simulink model "keshestatefeedback"  (R2017a)
settings: Solver=VariableStepAuto  StartTime=0.0  StopTime=10  MaxStep=0.01  RelTol=1e-3
settings Model: Creator=adi  LastModifiedBy=adi

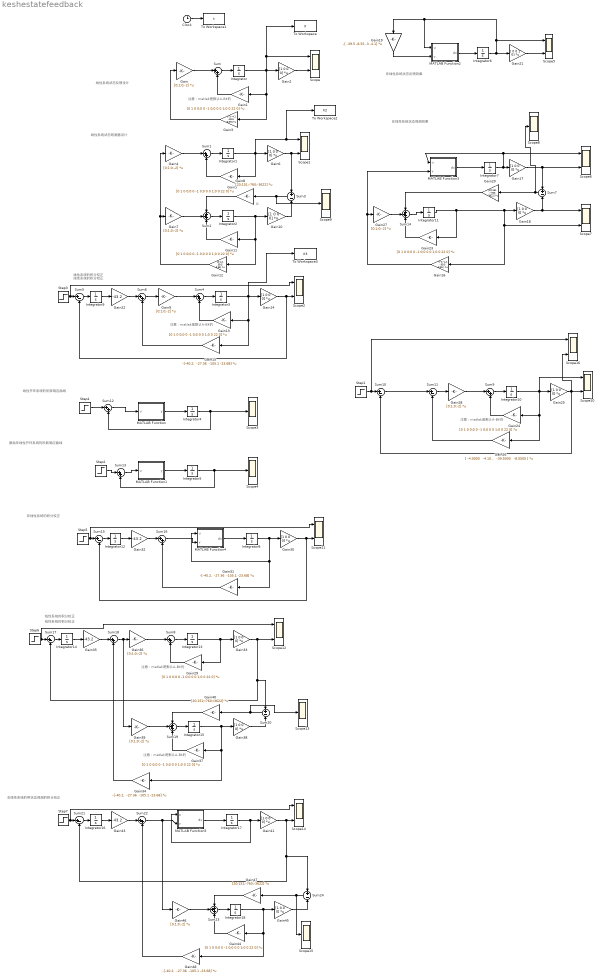
== system keshestatefeedback ==
  note: 非线性系统的积分校正
  note: 线性系统的积分校正
  note: G
  note: 线性系统状态反馈设计
  note: 线性开环系统的阶跃响应曲线
  note: 注意：matlab是默认A-BK的
  note: 注意：matlab是默认A-BK的
  note: 原始非线性开环系统的阶跃响应曲线
  note: 非线性系统状态反馈效果
  note: 非线性系统状态观测效果
  note: 线性系统状态观测器设计
  note: 注意：matlab是默认A-BK的
  note: 线性系统的积分校正
  note: 线性系统的积分校正
  note: 注意：matlab是默认A-BK的
  note: 线性系统的积分校正
  note: 注意：matlab是默认A-BK的
  note: 非线性系统的带状态观测的积分校正
  Clock : Clock
  Gain{,4,7,9,27..28,36,39,46} (9 alike) : Gain  Gain=[0;1;0;-2]  Multiplication=Matrix(K*u)
  Gain{1,5,11,13,23..24,29,37,44} (9 alike) : Gain  Gain=[0 1 0 0;0 0 -1 0;0 0 0 1;0 0 22 0]  Multiplication=Matrix(K*u)
  Gain{2,6,10,14,17..18,25,30,33,38,41,45} (12 alike) : Gain  Gain=[1 0 0 0]  Multiplication=Matrix(K*u)
  Gain12 : Gain  Gain=[3 4.1 39.5 8.55]  Multiplication=Matrix(K*u)
  Gain{15,31,34,48} (4 alike) : Gain  Gain="-[-40.2,  -27.36  -105.1 -23.68]"  Multiplication=Matrix(K*u)
  Gain16 : Gain  Gain="-[-3 -4.1 -39.5  -8.55 ]"  Multiplication=Matrix(K*u)
  Gain19 : Gain  Gain=-[ -39.5 -8.55 -3 -4.1]  Multiplication=Matrix(K*u)
  Gain20 : Gain  Gain="[20;151 ;-760;  -3622]"  Multiplication=Matrix(K*u)
  Gain21 : Gain  Gain=[ 0 0 1 0]  Multiplication=Matrix(K*u)
  Gain{22,32,35,43} (4 alike) : Gain  Gain=-43.2
  Gain26 : Gain  Gain=|  Multiplication=Matrix(K*u)
      | [ -4.0000   -4.1000  -39.5000   -8.5500
      | ]
  Gain3 : Gain  Gain=-[-3 -4.1 -39.5 -8.55]  Multiplication=Matrix(K*u)
  Gain40 : Gain  Gain=[20;151;-760;-3622]  Multiplication=Matrix(K*u)
  Gain47 : Gain  Gain=[20;151;-760;-3622]  Multiplication=Matrix(K*u)
  Gain8 : Gain  Gain=[20;151;-760;-3622]  Multiplication=Matrix(K*u)
  Integrator : Integrator  InitialCondition=[0.1 0 0 0]
  Integrator1 : Integrator  InitialCondition=[0.1 0 0 0]
  Integrator{3..5,8,10,13,15,17..18} (9 alike) : Integrator  InitialCondition=[0 0 0 0]
  Integrator11 : Integrator  InitialCondition=[0 0 0.1 0]
  Integrator{9,12,14,16} (4 alike) : Integrator
  Integrator2 : Integrator  InitialCondition=[0.001 0 0 0]
  Integrator6 : Integrator  InitialCondition=[0.1 0 0 0]
  Integrator7 : Integrator  InitialCondition=[0 0 0.1 0]
  MATLAB Function : MATLAB Function  TreatAsAtomicUnit=on
  MATLAB Function1 : MATLAB Function  TreatAsAtomicUnit=on
  MATLAB Function2 : MATLAB Function  TreatAsAtomicUnit=on
  MATLAB Function3 : MATLAB Function  TreatAsAtomicUnit=on
  MATLAB Function4 : MATLAB Function  TreatAsAtomicUnit=on
  MATLAB Function5 : MATLAB Function  TreatAsAtomicUnit=on
  Scope{,1..2,5..7,10..12,14,16} (11 alike) : Scope  NumInputPorts=2
  Scope{3..4,8..9,13,15} (6 alike) : Scope
  Step{1,3,5..7} (5 alike) : Step  After=0.1  SampleTime=0
  Step2 : Step  SampleTime=0
  Step4 : Step  SampleTime=0
  Sum{,1,4,6,8..9,12..13,16,18,22} (11 alike) : Sum  Inputs=|++
  Sum{5,10..11,15,17,21} (6 alike) : Sum  Inputs=|+-
  Sum{2,14,19,23} (4 alike) : Sum  Inputs=+++
  Sum{3,7,20,24} (4 alike) : Sum  Inputs=+-
  To Workspace : ToWorkspace  VariableName=X  SaveFormat=Structure With Time  SampleTime=-1
  To Workspace1 : ToWorkspace  VariableName=t  SaveFormat=Structure With Time  SampleTime=-1
  To Workspace2 : ToWorkspace  VariableName=X2  SaveFormat=Structure With Time  SampleTime=-1
  To Workspace3 : ToWorkspace  VariableName=X3  SaveFormat=Structure With Time  SampleTime=-1
  wires:
  Gain/1 -> Sum/1
  Sum/1 -> Integrator/1
  Integrator/1 -> To Workspace/1, Scope/1, Gain3/1, Gain1/1, Gain2/1
  Gain1/1 -> Sum/2
  Gain2/1 -> Scope/2
  Gain3/1 -> Gain/1
  Gain4/1 -> Sum1/1
  Sum1/1 -> Integrator1/1
  Gain5/1 -> Sum1/2
  Gain6/1 -> Sum3/1, Scope1/2
  Gain7/1 -> Sum2/2
  Sum2/1 -> Integrator2/1
  Gain10/1 -> Sum3/2
  Sum3/1 -> Scope9/1, Gain8/1
  Gain8/1 -> Sum2/1
  Gain11/1 -> Sum2/3
  Integrator2/1 -> Gain10/1, Gain12/1, Gain11/1
  Sum4/1 -> Integrator3/1
  Gain13/1 -> Sum4/2
  Gain15/1 -> Sum6/2
  Sum6/1 -> Gain9/1
  Gain12/1 -> Gain7/1, Gain4/1
  Clock/1 -> To Workspace1/1
  Integrator1/1 -> To Workspace2/1, Scope1/1, Gain5/1, Gain6/1
  Integrator3/1 -> To Workspace3/1, Gain15/1, Gain13/1, Gain14/1
  MATLAB Function/1(y) -> Integrator4/1
  Integrator4/1 -> Sum12/2, Scope3/1
  Integrator5/1 -> Sum13/2, Scope4/1
  MATLAB Function1/1(y) -> Integrator5/1
  MATLAB Function3/1(dx) -> Integrator7/1
  Integrator11/1 -> Gain23/1, Scope7/2, Gain16/1, Gain18/1
  Integrator7/1 -> MATLAB Function3/1(u), Scope6/1, Gain17/1
  Gain17/1 -> Sum7/1, Scope6/2
  Gain18/1 -> Sum7/2, Scope7/1
  Sum7/1 -> Scope8/1, Gain20/1
  Gain16/1 -> Gain27/1, MATLAB Function3/2(v)
  Integrator6/1 -> Gain21/1, Scope5/1, MATLAB Function2/1(u), Gain19/1
  MATLAB Function2/1(dx) -> Integrator6/1
  Gain19/1 -> MATLAB Function2/2(v)
  Gain21/1 -> Scope5/2
  Integrator9/1 -> Gain22/1
  Gain22/1 -> Sum6/1
  Gain25/1 -> Scope16/2, Sum10/2, Scope10/2
  Gain24/1 -> Sum9/2
  Sum9/1 -> Integrator10/1
  Integrator10/1 -> Scope10/1, Gain26/1, Gain24/1, Gain25/1
  Sum11/1 -> Gain28/1
  Gain28/1 -> Sum9/1
  Step1/1 -> Scope16/1, Sum10/1
  Gain26/1 -> Sum11/2
  Sum10/1 -> Sum11/1
  Sum5/1 -> Integrator9/1
  Step3/1 -> Scope2/1, Sum5/1
  Gain14/1 -> Sum5/2, Scope2/2
  Step4/1 -> Sum12/1
  Sum12/1 -> MATLAB Function/1(u)
  Gain9/1 -> Sum4/1
  Step2/1 -> Sum13/1
  Sum13/1 -> MATLAB Function1/1(u)
  Sum14/1 -> Integrator11/1
  Gain23/1 -> Sum14/3
  Gain27/1 -> Sum14/2
  Gain20/1 -> Sum14/1
  Integrator12/1 -> Gain32/1
  Gain30/1 -> Sum15/2, Scope11/2
  Gain31/1 -> Sum16/2
  Gain32/1 -> Sum16/1
  Step5/1 -> Scope11/1, Sum15/1
  Sum15/1 -> Integrator12/1
  Sum16/1 -> MATLAB Function4/2(v)
  MATLAB Function4/1(dx) -> Integrator8/1
  Integrator8/1 -> Gain31/1, MATLAB Function4/1(u), Gain30/1
  Sum8/1 -> Integrator13/1
  Gain29/1 -> Sum8/2
  Gain36/1 -> Sum8/1
  Integrator14/1 -> Gain35/1
  Gain34/1 -> Sum18/2
  Gain35/1 -> Sum18/1
  Integrator13/1 -> Gain29/1, Gain33/1
  Step6/1 -> Scope12/1, Sum17/1
  Sum18/1 -> Gain39/1, Gain36/1
  Sum17/1 -> Integrator14/1
  Integrator15/1 -> Gain34/1, Gain37/1, Gain38/1
  Sum19/1 -> Integrator15/1
  Gain39/1 -> Sum19/2
  Gain37/1 -> Sum19/3
  Gain33/1 -> Sum20/1, Sum17/2, Scope12/2
  Gain38/1 -> Sum20/2
  Sum20/1 -> Scope13/1, Gain40/1
  Gain40/1 -> Sum19/1
  Integrator17/1 -> MATLAB Function5/1(u), Gain41/1
  MATLAB Function5/1(dx) -> Integrator17/1
  Sum22/1 -> Gain46/1, MATLAB Function5/2(v)
  Step7/1 -> Scope14/1, Sum21/1
  Sum21/1 -> Integrator16/1
  Integrator16/1 -> Gain43/1
  Gain43/1 -> Sum22/1
  Sum24/1 -> Gain47/1, Scope15/1
  Gain44/1 -> Sum23/3
  Gain45/1 -> Sum24/2
  Sum23/1 -> Integrator18/1
  Gain47/1 -> Sum23/1
  Integrator18/1 -> Gain48/1, Gain44/1, Gain45/1
  Gain46/1 -> Sum23/2
  Gain41/1 -> Sum24/1, Sum21/2, Scope14/2
  Gain48/1 -> Sum22/2

== matlab function keshestatefeedback/MATLAB Function1 ==
  data: u input; y output
function y = fcn(u)
M=1;m=0.1;l=0.5;g=9.8;v=0;
dx1 = u(2);
dx2 = (v*cos(u(1))-(M+m)*g*sin(u(1))+m*l*sin(u(1))*cos(u(1)*u(2)*u(2)))/(m*l*cos(u(1))*cos(u(1))-(M+m)*l);
dx3 = u(4);
dx4 = (v+m*l*sin(u(1)*u(2)*u(2))-m*g*cos(u(1))*sin(u(1)))/(M+m-m*cos(u(1))*cos(u(1)));
y = [dx1;dx2;dx3;dx4];

== matlab function keshestatefeedback/MATLAB Function ==
  data: u input; y output
function y = fcn(u)
M=1;m=0.1;l=0.5;g=9.8;v=0;
dx1 = u(2);
dx2 = (-1*m*g/M)*u(3)+(1/M)*v;
dx3 = u(4);
dx4 = ((M+m)*g/M/l)*u(3)-(1/M/l)*v;
y = [dx1;dx2;dx3;dx4];

== matlab function keshestatefeedback/MATLAB Function2 ==
  data: dx output; u input; v input
function dx = fcn(u,v)
M=1;m=0.1;l=0.5;g=10;
%v=0;
dx1 = u(2);
dx2=(v*cos(u(1))-(M+m)*g*sin(u(1))+m*l*sin(u(1))*cos(u(1))*u(2)*u(2))/(m*l*cos(u(1))*cos(u(1))-(M+m)*l);
%dx2 = (v*cos(u(1))-(M+m)*g*sin(u(1))+m*l*sin(u(1))*cos((u(1))*u(2)*u(2)))/(m*l*cos(u(1))*cos(u(1))-(M+m)*l);
dx3 = u(4);
dx4 = (v+m*l*sin(u(1)*u(2)*u(2))-m*g*cos(u(1))*sin(u(1)))/(M+m-m*cos(u(1))*cos(u(1)));
dx = [dx1;dx2;dx3;dx4];

== matlab function keshestatefeedback/MATLAB Function3 ==
  data: u input; dx output; v input
function dx = fcn(u,v)
M=1;m=0.1;l=0.5;g=9.8;
%v=0;
dx1 = u(2);
dx4 = (v*cos(u(3))-(M+m)*g*sin(u(3))+m*l*sin(u(3))*cos(u(3)*u(4)*u(4)))/(m*l*cos(u(3))*cos(u(3))-(M+m)*l);
dx3 = u(4);
dx2= (v+m*l*sin(u(3)*u(4)*u(4))-m*g*cos(u(3))*sin(u(3)))/(M+m-m*cos(u(3))*cos(u(3)));
dx = [dx1;dx2;dx3;dx4];

== matlab function keshestatefeedback/MATLAB Function4 ==
  data: u input; dx output; v input
function dx = fcn(u,v)
M=1;m=0.1;l=0.5;g=9.8;
%v=0;
dx1 = u(2);
dx4 = (v*cos(u(3))-(M+m)*g*sin(u(3))+m*l*sin(u(3))*cos(u(3)*u(4)*u(4)))/(m*l*cos(u(3))*cos(u(3))-(M+m)*l);
dx3 = u(4);
dx2= (v+m*l*sin(u(3)*u(4)*u(4))-m*g*cos(u(3))*sin(u(3)))/(M+m-m*cos(u(3))*cos(u(3)));
dx = [dx1;dx2;dx3;dx4];

== matlab function keshestatefeedback/MATLAB Function5 ==
  data: u input; dx output; v input
function dx = fcn(u,v)
M=1;m=0.1;l=0.5;g=9.8;
%v=0;
dx1 = u(2);
dx4 = (v*cos(u(3))-(M+m)*g*sin(u(3))+m*l*sin(u(3))*cos(u(3)*u(4)*u(4)))/(m*l*cos(u(3))*cos(u(3))-(M+m)*l);
dx3 = u(4);
dx2= (v+m*l*sin(u(3)*u(4)*u(4))-m*g*cos(u(3))*sin(u(3)))/(M+m-m*cos(u(3))*cos(u(3)));
dx = [dx1;dx2;dx3;dx4];
